simulink model "SWC_SWD"  (R2020a)
settings: Solver=FixedStepDiscrete  StartTime=0.0  StopTime=1  FixedStep=0.0001  RelTol=1e-3
undefined symbols (not defined in the file): CAL_SWD_AgrslvCompCnt_f32, CAL_SWD_MotorPole_u8, CAL_SWD_Radian_u16, GLB_SWD_CircAge_f32, GLB_SWD_MotorPole_u8, GLB_SWD_OneHalf_f32, GLB_SWD_pi_f32, GLB_SWD_Sixty_f32
libraries: simulink x5
settings Model: DataDictionary=SWC_SWD_DataDictionary.sldd  Creator=dongliyuan  LastModifiedBy=wangqianglong
settings DataIOCC: SaveFormat=StructureWithTime
settings OptimizationCC: DefaultParameterBehavior=Inlined  EnhancedBackFolding=on  PassReuseOutputArgsAs=Individual arguments  ZeroExternalMemoryAtStartup=off  ZeroInternalMemoryAtStartup=off  OptimizeBlockOrder=speed  DifferentSizesBufferReuse=on  OptimizationCustomize=off  EfficientTunableParamExpr=on
settings DebuggingCC: SignalInfNanChecking=warning  ParameterPrecisionLossMsg=none  ParameterTunabilityLossMsg=error  UnnecessaryDatatypeConvMsg=warning  VectorMatrixConversionMsg=warning  StrictBusMsg=WarnOnBusTreatedAsVector  NonBusSignalsTreatedAsBus=warning
settings ModelReferenceCC: ModelReferenceNumInstancesAllowed=Single
settings SFSimCC: MATLABDynamicMemAlloc=off
settings RTWCC: SystemTargetFile=ert.tlc  GenCodeOnly=on  TemplateMakefile=ert_default_tmf  CustomSourceCode="#include \"set_get_data.h\""
settings CodeAppCC: ForceParamTrailComments=on  IgnoreCustomStorageClasses=off  OperatorAnnotations=on  SimulinkDataObjDesc=on  SFDataObjDesc=on  InsertBlockDesc=on
settings ERTTargetCC: TargetLangStandard=C99 (ISO)  UtilityFuncGeneration=Shared location  GenerateASAP2=on  InlinedParameterPlacement=NonHierarchical  ERTCustomFileTemplate=example_file_process.tlc  EnableUserReplacementTypes=on

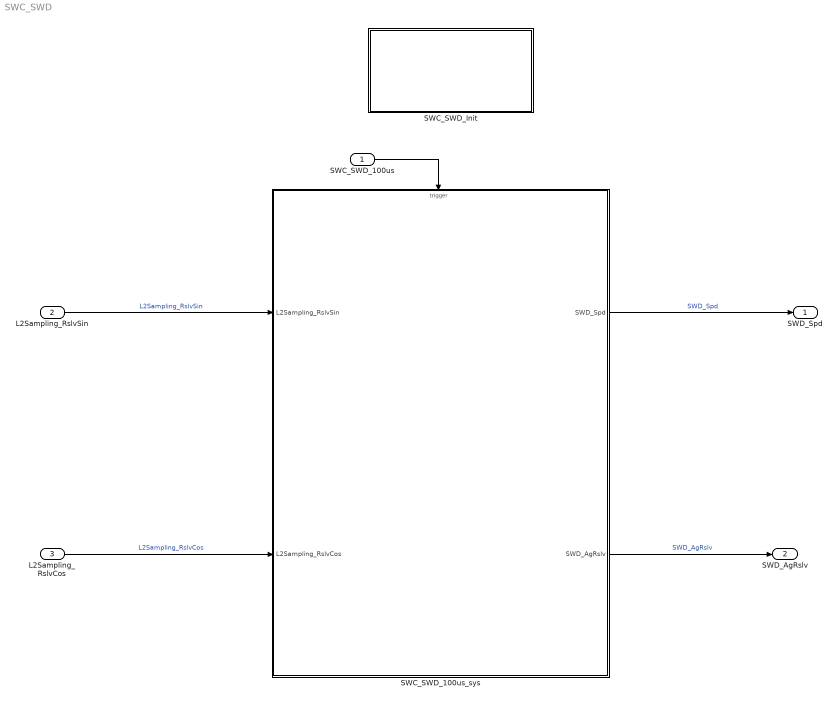
== system SWC_SWD ==
  SWC_SWD_100us : Inport  SampleTime=0.0001  OutputFunctionCall=on
  L2Sampling_RslvSin : Inport  Port=2  OutDataTypeStr=single  PortDimensions=1
  L2Sampling_RslvCos : Inport  Port=3  OutDataTypeStr=single  PortDimensions=1
  SWC_SWD_100us_sys : Subsystem
  SWC_SWD_Init : Subsystem
  SWD_Spd : Outport  VectorParamsAs1DForOutWhenUnconnected=off
  SWD_AgRslv : Outport  Port=2  VectorParamsAs1DForOutWhenUnconnected=off
  wires:
  L2Sampling_RslvSin/1 -> SWC_SWD_100us_sys/1(L2Sampling_RslvSin)  "L2Sampling_RslvSin"
  SWC_SWD_100us/1 -> SWC_SWD_100us_sys/Trigger
  L2Sampling_RslvCos/1 -> SWC_SWD_100us_sys/2(L2Sampling_RslvCos)  "L2Sampling_RslvCos"
  SWC_SWD_100us_sys/1(SWD_Spd) -> SWD_Spd/1  "SWD_Spd"
  SWC_SWD_100us_sys/2(SWD_AgRslv) -> SWD_AgRslv/1  "SWD_AgRslv"

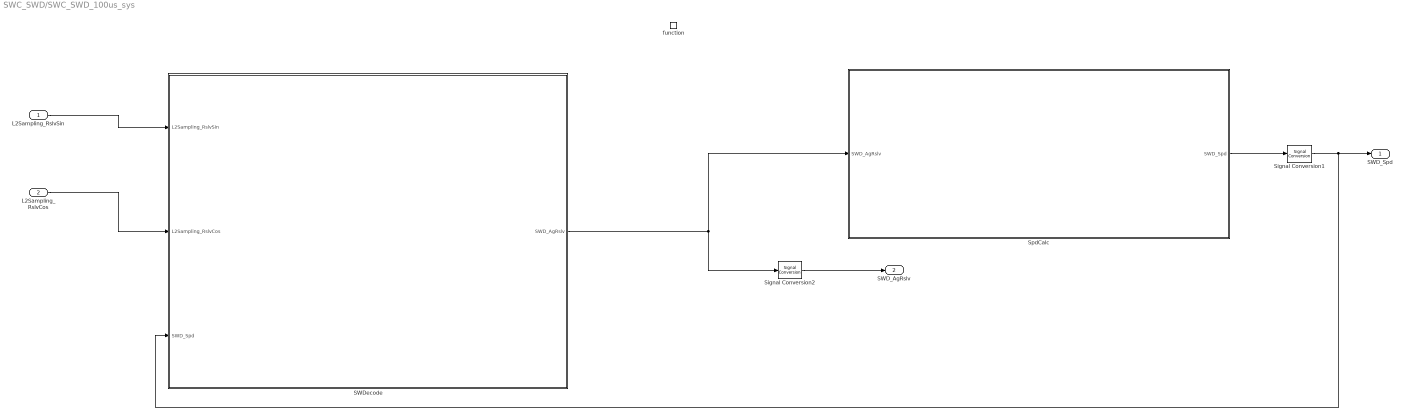
== system SWC_SWD/SWC_SWD_100us_sys ==
  L2Sampling_RslvSin : Inport
  L2Sampling_RslvCos : Inport  Port=2
  function : TriggerPort  TriggerType=function-call  VariantControl=(inherit)  SampleTimeType=periodic  SampleTime=-1
  SWDecode : Subsystem
  Signal Conversion1 : SignalConversion  OverrideOpt=off
  Signal Conversion2 : SignalConversion  OverrideOpt=off
  SpdCalc : Subsystem
  SWD_Spd : Outport  VectorParamsAs1DForOutWhenUnconnected=off
  SWD_AgRslv : Outport  Port=2  VectorParamsAs1DForOutWhenUnconnected=off
  wires:
  L2Sampling_RslvSin/1 -> SWDecode/1(L2Sampling_RslvSin)
  L2Sampling_RslvCos/1 -> SWDecode/2(L2Sampling_RslvCos)
  SpdCalc/1(SWD_Spd) -> Signal Conversion1/1
  SWDecode/1(SWD_AgRslv) -> Signal Conversion2/1, SpdCalc/1(SWD_AgRslv)
  Signal Conversion1/1 -> SWDecode/3(SWD_Spd), SWD_Spd/1
  Signal Conversion2/1 -> SWD_AgRslv/1

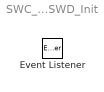
== system SWC_SWD/SWC_SWD_Init ==
  Event Listener : EventListener  EventName=reset

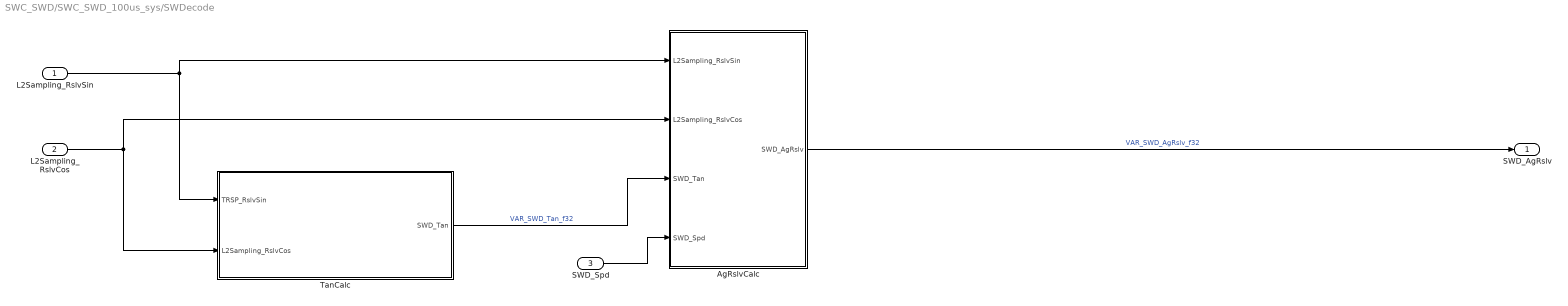
== system SWC_SWD/SWC_SWD_100us_sys/SWDecode ==
  L2Sampling_RslvSin : Inport
  L2Sampling_RslvCos : Inport  Port=2
  SWD_Spd : Inport  Port=3
  AgRslvCalc : Subsystem  TreatAsAtomicUnit=on
      settings: RTWSystemCode=Nonreusable function
  TanCalc : Subsystem  TreatAsAtomicUnit=on
      settings: RTWSystemCode=Nonreusable function
  SWD_AgRslv : Outport  VectorParamsAs1DForOutWhenUnconnected=off
  wires:
  AgRslvCalc/1(SWD_AgRslv) -> SWD_AgRslv/1  "VAR_SWD_AgRslv_f32"
  L2Sampling_RslvCos/1 -> TanCalc/2(L2Sampling_RslvCos), AgRslvCalc/2(L2Sampling_RslvCos)
  L2Sampling_RslvSin/1 -> TanCalc/1(TRSP_RslvSin), AgRslvCalc/1(L2Sampling_RslvSin)
  TanCalc/1(SWD_Tan) -> AgRslvCalc/3(SWD_Tan)  "VAR_SWD_Tan_f32"
  SWD_Spd/1 -> AgRslvCalc/4(SWD_Spd)

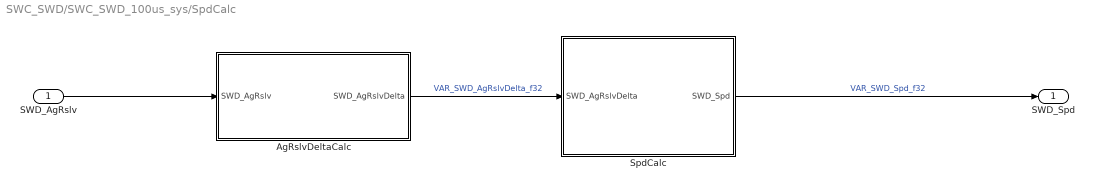
== system SWC_SWD/SWC_SWD_100us_sys/SpdCalc ==
  SWD_AgRslv : Inport
  AgRslvDeltaCalc : Subsystem  TreatAsAtomicUnit=on
      settings: RTWSystemCode=Nonreusable function
  SpdCalc : Subsystem  TreatAsAtomicUnit=on
      settings: RTWSystemCode=Nonreusable function
  SWD_Spd : Outport  VectorParamsAs1DForOutWhenUnconnected=off
  wires:
  AgRslvDeltaCalc/1(SWD_AgRslvDelta) -> SpdCalc/1(SWD_AgRslvDelta)  "VAR_SWD_AgRslvDelta_f32"
  SpdCalc/1(SWD_Spd) -> SWD_Spd/1  "VAR_SWD_Spd_f32"
  SWD_AgRslv/1 -> AgRslvDeltaCalc/1(SWD_AgRslv)

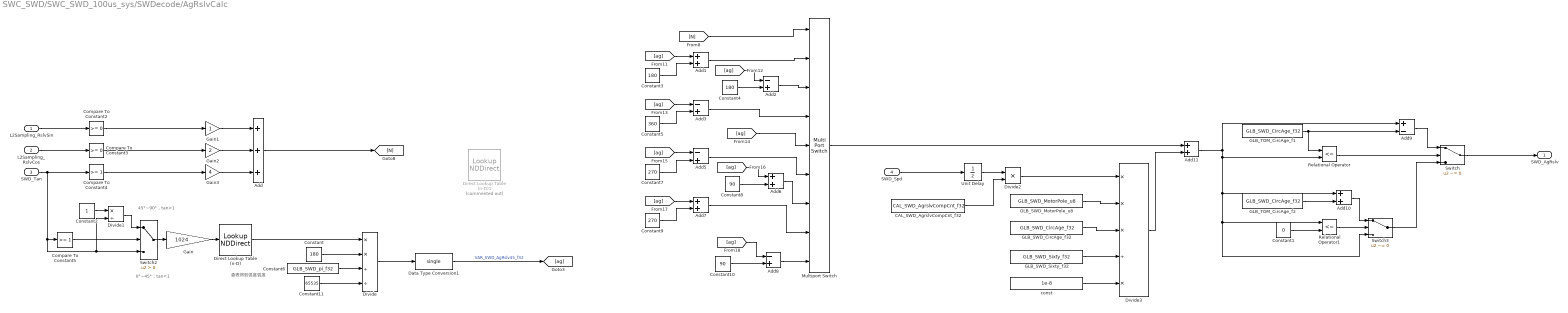
== system SWC_SWD/SWC_SWD_100us_sys/SWDecode/AgRslvCalc ==
  note: 0°~45°，tan<1
  note: 45°~90°，tan>1
  note: 查表得到弧度弧度
  L2Sampling_RslvSin : Inport
  L2Sampling_RslvCos : Inport  Port=2
  SWD_Tan : Inport  Port=3
  SWD_Spd : Inport  Port=4
  Add : Sum  Inputs=+++
  Add{1,6..7,10..11} (5 alike) : Sum
  Add{2..3,5,8} (4 alike) : Sum  Inputs=-+
  Add9 : Sum  Inputs=+-
  CAL_SWD_AgrslvCompCnt_f32 : Constant  Value=CAL_SWD_AgrslvCompCnt_f32  OutDataTypeStr=single
  Compare To Constant2 : simulink/Logic and Bit Operations/Compare To Constant  relop=>=  const=0  OutDataTypeStr=uint8
  Compare To Constant3 : simulink/Logic and Bit Operations/Compare To Constant  relop=>=  const=0  OutDataTypeStr=uint8
  Compare To Constant4 : simulink/Logic and Bit Operations/Compare To Constant  relop=>=  const=1  OutDataTypeStr=uint8
  Compare To Constant5 : simulink/Logic and Bit Operations/Compare To Constant  relop=>=  const=1  OutDataTypeStr=boolean
  Constant : Constant  Value=180  OutDataTypeStr=single
  Constant1 : Constant  Value=0  OutDataTypeStr=single
  Constant10 : Constant  Value=90  OutDataTypeStr=single
  Constant11 : Constant  Value=65535  OutDataTypeStr=single
  Constant2 : Constant  OutDataTypeStr=single
  Constant3 : Constant  Value=180  OutDataTypeStr=single
  Constant4 : Constant  Value=180  OutDataTypeStr=single
  Constant5 : Constant  Value=360  OutDataTypeStr=single
  Constant6 : Constant  Value=GLB_SWD_pi_f32
  Constant7 : Constant  Value=270  OutDataTypeStr=single
  Constant8 : Constant  Value=90  OutDataTypeStr=single
  Constant9 : Constant  Value=270  OutDataTypeStr=single
  Data Type Conversion1 : DataTypeConversion  OutDataTypeStr=single
  Direct Lookup Table (n-D) : LookupNDDirect  NumberOfTableDimensions=1  Table=CAL_SWD_Radian_u16  RemoveProtectionInput=on  TableDataTypeStr=uint16
  Direct Lookup Table (n-D)1 : LookupNDDirect  Commented=on  NumberOfTableDimensions=1  Table="[0\t64\t128\t192\t256\t320\t384\t448\t512\t576\t640\t704\t768\t832\t896\t960\t1024\t1088\t1152\t1216\t1280\t1344\t1408\t1472\t1536\t1600\t1664\t1728\t1792\t1855\t1919\t1983\t2047\t2111\t2175\t2239\t2303\t2367\t2431\t2495\t2559\t2623\t2686\t2750\t2814\t2878\t2942\t3006\t3070\t3134\t3197\t3261\t3325\t3389\t3453\t3517\t3580\t3644\t3708\t3772\t3836\t3899\t3963\t4027\t4091\t4154\t4218\t4282\t4346\t4409 ...(+6597 chars)]"  TableDataTypeStr=uint16
  Divide : Product  Inputs=**//
  Divide1 : Product  Inputs=*/
  Divide2 : Product  Inputs=**
  Divide3 : Product  Inputs=***/*
  GLB_SWD_CircAge_f32 : Constant  Value=GLB_SWD_CircAge_f32  OutDataTypeStr=single
  GLB_SWD_MotorPole_u8 : Constant  Value=GLB_SWD_MotorPole_u8  OutDataTypeStr=single
  GLB_SWD_Sixty_f32 : Constant  Value=GLB_SWD_Sixty_f32  OutDataTypeStr=single
  GLB_TOM_CircAge_f1 : Constant  Value=GLB_SWD_CircAge_f32
  GLB_TOM_CircAge_f2 : Constant  Value=GLB_SWD_CircAge_f32
  Gain : Gain  Gain=1024
  Gain1 : Gain  OutDataTypeStr=uint8
  Gain2 : Gain  Gain=2  OutDataTypeStr=uint8
  Gain3 : Gain  Gain=4  OutDataTypeStr=uint8
  Multiport Switch : MultiPortSwitch  DataPortOrder=Zero-based contiguous  Inputs=8  zeroidx=on
  Relational Operator : RelationalOperator  Operator=<=  OutDataTypeStr=boolean  RndMeth=Simplest
  Relational Operator1 : RelationalOperator  Operator=<=  OutDataTypeStr=boolean  RndMeth=Simplest
  Switch : Switch  Criteria=u2 ~= 0
  Switch2 : Switch  Criteria=u2 > Threshold
  Switch3 : Switch  Criteria=u2 ~= 0
  Unit Delay : UnitDelay  SampleTime=-1  HasFrameUpgradeWarning=on
  const : Constant  Value=1e-8  OutDataTypeStr=single
  SWD_AgRslv : Outport
  wires:
  [ag] -> Add3/1
  [ag] -> Add5/1
  Compare To Constant2/1 -> Gain1/1
  [ag] -> Add1/1
  Constant4/1 -> Add2/2
  Constant10/1 -> Add8/2
  Add7/1 -> Multiport Switch/8
  Gain3/1 -> Add/3
  [ag] -> Add7/1
  L2Sampling_RslvCos/1 -> Compare To Constant3/1
  Constant9/1 -> Add7/2
  L2Sampling_RslvSin/1 -> Compare To Constant2/1
  Add8/1 -> Multiport Switch/9
  Gain1/1 -> Add/1
  [ag] -> Add6/1
  Add6/1 -> Multiport Switch/7
  [ag] -> Multiport Switch/5
  Add1/1 -> Multiport Switch/2
  Add5/1 -> Multiport Switch/6
  [ag] -> Add2/1
  Compare To Constant4/1 -> Gain3/1
  Constant7/1 -> Add5/2
  Add2/1 -> Multiport Switch/3
  Constant5/1 -> Add3/2
  Add3/1 -> Multiport Switch/4
  Constant8/1 -> Add6/2
  [ag] -> Add8/1
  Gain2/1 -> Add/2
  Compare To Constant3/1 -> Gain2/1
  Constant3/1 -> Add1/2
  [N] -> Multiport Switch/1
  Switch2/1 -> Gain/1
  Constant2/1 -> Divide1/1
  Divide1/1 -> Switch2/1
  Direct Lookup Table (n-D)/1 -> Divide/1
  SWD_Tan/1 -> Compare To Constant4/1, Divide1/2, Switch2/3, Compare To Constant5/1
  Gain/1 -> Direct Lookup Table (n-D)/1
  Compare To Constant5/1 -> Switch2/2
  Constant6/1 -> Divide/3
  Constant/1 -> Divide/2
  Constant11/1 -> Divide/4
  Divide/1 -> Data Type Conversion1/1
  Add/1 -> [N]
  Data Type Conversion1/1 -> [ag]  "VAR_SWD_AgRslv45_f32"
  Multiport Switch/1 -> Add11/1
  Divide2/1 -> Divide3/1
  Unit Delay/1 -> Divide2/1
  Switch3/1 -> Switch/3
  Constant1/1 -> Relational Operator1/2
  Relational Operator/1 -> Switch/2
  Add10/1 -> Switch3/1
  Switch/1 -> SWD_AgRslv/1
  GLB_TOM_CircAge_f2/1 -> Add10/2
  Relational Operator1/1 -> Switch3/2
  Add9/1 -> Switch/1
  Add11/1 -> Add10/1, Relational Operator1/1, Switch3/3, Relational Operator/2, Add9/1
  GLB_TOM_CircAge_f1/1 -> Add9/2, Relational Operator/1
  Divide3/1 -> Add11/2
  SWD_Spd/1 -> Unit Delay/1
  CAL_SWD_AgrslvCompCnt_f32/1 -> Divide2/2
  GLB_SWD_MotorPole_u8/1 -> Divide3/2
  GLB_SWD_CircAge_f32/1 -> Divide3/3
  GLB_SWD_Sixty_f32/1 -> Divide3/4
  const/1 -> Divide3/5

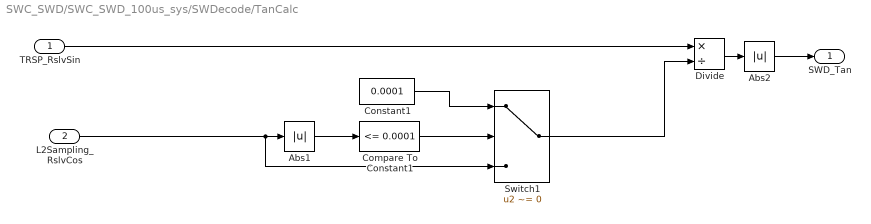
== system SWC_SWD/SWC_SWD_100us_sys/SWDecode/TanCalc ==
  TRSP_RslvSin : Inport
  L2Sampling_RslvCos : Inport  Port=2
  Abs1 : Abs
  Abs2 : Abs
  Compare To Constant1 : simulink/Logic and Bit Operations/Compare To Constant  relop=<=  const=0.0001  OutDataTypeStr=boolean
  Constant1 : Constant  Value=0.0001  OutDataTypeStr=single
  Divide : Product  Inputs=*/
  Switch1 : Switch  Criteria=u2 ~= 0
  SWD_Tan : Outport
  wires:
  Constant1/1 -> Switch1/1
  TRSP_RslvSin/1 -> Divide/1
  L2Sampling_RslvCos/1 -> Abs1/1, Switch1/3
  Switch1/1 -> Divide/2
  Compare To Constant1/1 -> Switch1/2
  Abs1/1 -> Compare To Constant1/1
  Abs2/1 -> SWD_Tan/1
  Divide/1 -> Abs2/1

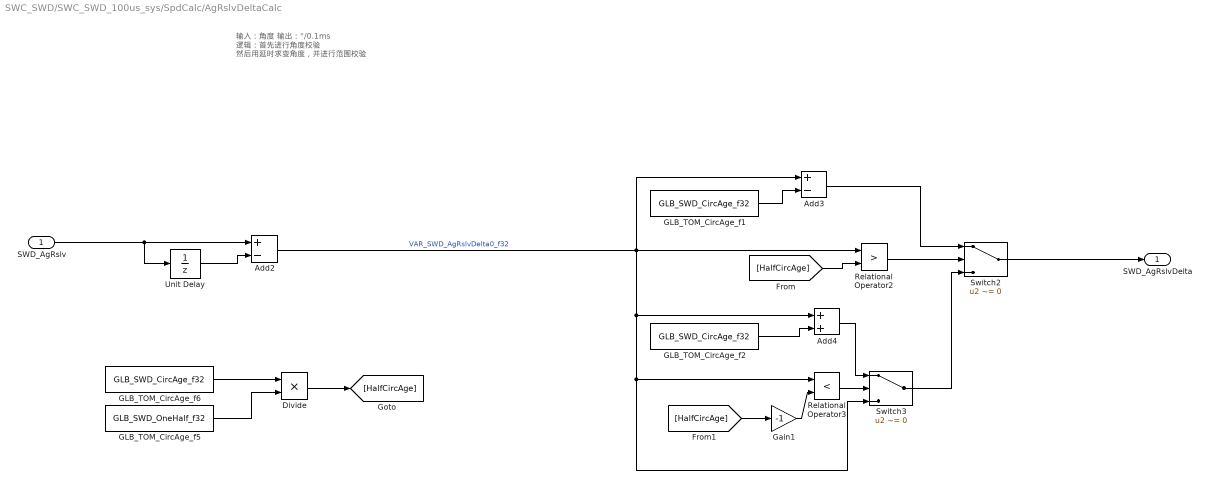
== system SWC_SWD/SWC_SWD_100us_sys/SpdCalc/AgRslvDeltaCalc ==
  note: 输入：角度
      | 输出：°/0.1ms
      | 逻辑：首先进行角度校验
      | 然后用延时求变角度，并进行范围校验
  SWD_AgRslv : Inport
  Add2 : Sum  Inputs=+-
  Add3 : Sum  Inputs=+-
  Add4 : Sum
  Divide : Product  Inputs=**
  GLB_TOM_CircAge_f1 : Constant  Value=GLB_SWD_CircAge_f32
  GLB_TOM_CircAge_f2 : Constant  Value=GLB_SWD_CircAge_f32
  GLB_TOM_CircAge_f5 : Constant  Value=GLB_SWD_OneHalf_f32
  GLB_TOM_CircAge_f6 : Constant  Value=GLB_SWD_CircAge_f32
  Gain1 : Gain  Gain=-1  OutDataTypeStr=single
  Relational Operator2 : RelationalOperator  Operator=>  OutDataTypeStr=boolean  RndMeth=Simplest
  Relational Operator3 : RelationalOperator  Operator=<  OutDataTypeStr=boolean  RndMeth=Simplest
  Switch2 : Switch  Criteria=u2 ~= 0
  Switch3 : Switch  Criteria=u2 ~= 0
  Unit Delay : UnitDelay  SampleTime=-1  HasFrameUpgradeWarning=on
  SWD_AgRslvDelta : Outport  VectorParamsAs1DForOutWhenUnconnected=off
  wires:
  [HalfCircAge] -> Gain1/1
  [HalfCircAge] -> Relational Operator2/2
  Divide/1 -> [HalfCircAge]
  GLB_TOM_CircAge_f5/1 -> Divide/2
  GLB_TOM_CircAge_f6/1 -> Divide/1
  Gain1/1 -> Relational Operator3/2
  Add3/1 -> Switch2/1
  Relational Operator3/1 -> Switch3/2
  Switch3/1 -> Switch2/3
  Relational Operator2/1 -> Switch2/2
  GLB_TOM_CircAge_f2/1 -> Add4/2
  Add4/1 -> Switch3/1
  Unit Delay/1 -> Add2/2
  GLB_TOM_CircAge_f1/1 -> Add3/2
  SWD_AgRslv/1 -> Unit Delay/1, Add2/1
  Add2/1 -> Add3/1, Switch3/3, Relational Operator3/1, Add4/1, Relational Operator2/1  "VAR_SWD_AgRslvDelta0_f32"
  Switch2/1 -> SWD_AgRslvDelta/1

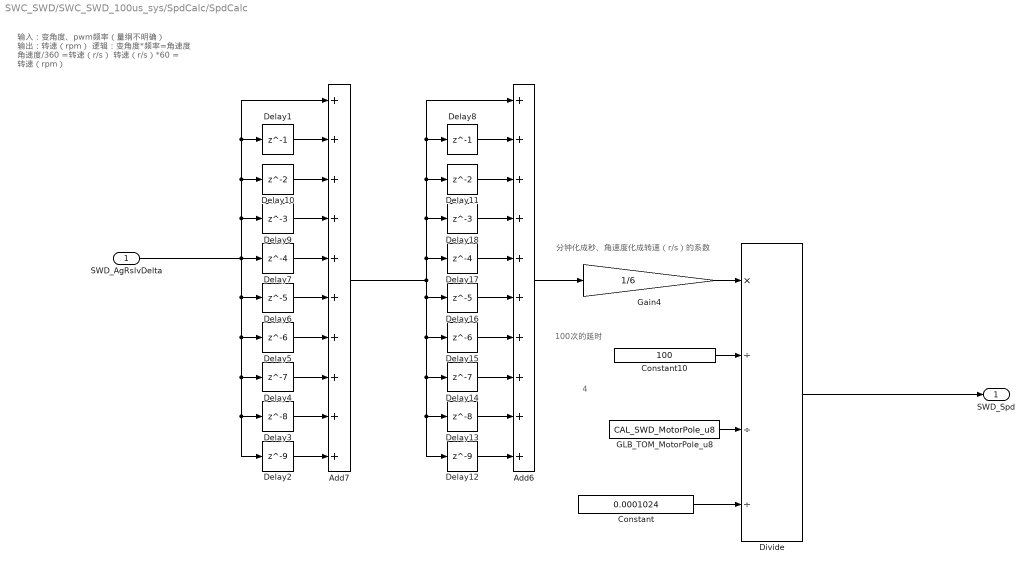
== system SWC_SWD/SWC_SWD_100us_sys/SpdCalc/SpdCalc ==
  note: 4
  note: 100次的延时
  note: 输入：变角度、pwm频率（量纲不明确）
      | 输出：转速（rpm）
      |
      | 逻辑：变角度*频率=角速度
      | 角速度/360 =转速（r/s）
      | 转速（r/s）*60 = 转速（rpm）
  note: 分钟化成秒、角速度化成转速（r/s）的系数
  SWD_AgRslvDelta : Inport
  Add6 : Sum  Inputs=++++++++++
  Add7 : Sum  Inputs=++++++++++
  Constant : Constant  Value=0.0001024  OutDataTypeStr=single
  Constant10 : Constant  Value=100  OutDataTypeStr=uint8
  Delay1 : Delay  DelayLength=1
  Delay10 : Delay
  Delay11 : Delay
  Delay12 : Delay  DelayLength=9
  Delay13 : Delay  DelayLength=8
  Delay14 : Delay  DelayLength=7
  Delay15 : Delay  DelayLength=6
  Delay16 : Delay  DelayLength=5
  Delay17 : Delay  DelayLength=4
  Delay18 : Delay  DelayLength=3
  Delay2 : Delay  DelayLength=9
  Delay3 : Delay  DelayLength=8
  Delay4 : Delay  DelayLength=7
  Delay5 : Delay  DelayLength=6
  Delay6 : Delay  DelayLength=5
  Delay7 : Delay  DelayLength=4
  Delay8 : Delay  DelayLength=1
  Delay9 : Delay  DelayLength=3
  Divide : Product  Inputs=*///
  GLB_TOM_MotorPole_u8 : Constant  Value=CAL_SWD_MotorPole_u8
  Gain4 : Gain  Gain=1/6
  SWD_Spd : Outport  VectorParamsAs1DForOutWhenUnconnected=off
  wires:
  Divide/1 -> SWD_Spd/1
  Delay5/1 -> Add7/7
  Delay11/1 -> Add6/3
  Delay17/1 -> Add6/5
  Delay16/1 -> Add6/6
  Delay14/1 -> Add6/8
  Delay12/1 -> Add6/10
  Delay8/1 -> Add6/2
  Add7/1 -> Delay12/1, Delay13/1, Delay14/1, Delay15/1, Delay16/1, Delay17/1, Delay18/1, Delay11/1, Delay8/1, Add6/1
  Add6/1 -> Gain4/1
  Delay13/1 -> Add6/9
  Delay10/1 -> Add7/3
  Delay9/1 -> Add7/4
  Delay7/1 -> Add7/5
  Delay6/1 -> Add7/6
  Delay18/1 -> Add6/4
  Delay15/1 -> Add6/7
  GLB_TOM_MotorPole_u8/1 -> Divide/3
  Constant10/1 -> Divide/2
  Delay4/1 -> Add7/8
  Delay3/1 -> Add7/9
  Gain4/1 -> Divide/1
  Delay2/1 -> Add7/10
  Delay1/1 -> Add7/2
  SWD_AgRslvDelta/1 -> Delay2/1, Delay3/1, Delay4/1, Delay5/1, Delay6/1, Delay9/1, Delay10/1, Delay1/1, Add7/1, Delay7/1
  Constant/1 -> Divide/4
